simulink model "delay_plant_2015B"  (R2015b)
settings: Solver=VariableStepAuto  StartTime=0.0  StopTime=sim_run  FixedStep=0.0001  RelTol=1e-3
undefined symbols (not defined in the file): DiscIntNeverNeededParam, Standard_Devices, start_packet_test, UDP_Protocol, zh_step
libraries: sldrtlib x2, simulink x1, dspnetwork x1
settings Model: Creator=Anony  LastModifiedBy=Anony

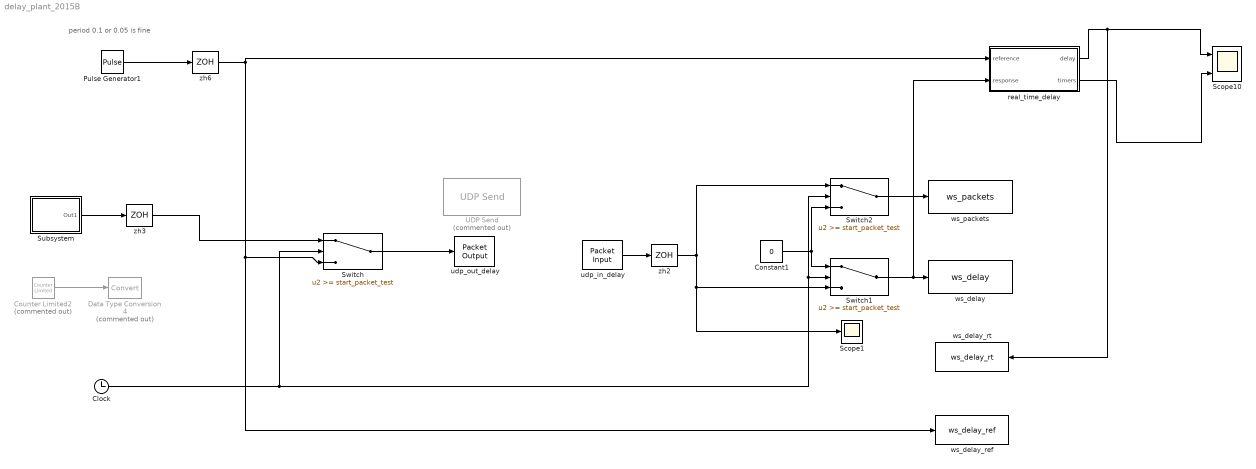
== system delay_plant_2015B ==
  note: period 0.1 or 0.05 is fine
  Clock : Clock
  Constant1 : Constant  Value=0
  Counter Limited2 : simulink/Sources/Counter Limited  Commented=on  uplimit=9999  tsamp=0.001
  Data Type Conversion4 : DataTypeConversion  Commented=on
  Pulse Generator1 : DiscretePulseGenerator  PulseType=Time based  Period=0.5  PulseWidth=0.000001
  Scope1 : Scope
  Scope10 : Scope  NumInputPorts=2
  Subsystem : Subsystem
  Switch : Switch  Threshold=start_packet_test
  Switch1 : Switch  Threshold=start_packet_test
  Switch2 : Switch  Threshold=start_packet_test
  UDP Send : dspnetwork/UDP Send  Commented=on  remoteURL='127.0.0.1'  remotePort=25000  localURL='0.0.0.0'  localPortSource=Automatically determine  localPort=-1  sampletime=-1  separateLengthPort=0
  real_time_delay : Subsystem
  udp_in_delay : sldrtlib/Packet Input  SampleTime=0.0001  MaxMissedTicks=inf  ShowMissedTicks=off  YieldWhenWaiting=off  DrvName=Standard_Devices/UDP_Protocol  DrvAddress=27000  DrvOptions=[2468394752 27000]  PacketSize=8  DataTypes='double'  ShowReady=off  ShowError=off  PacketID=1  ByteOrder=1  ShowTimestamp=off
      settings: AttributesFormatString=Standard Devices\nUDP Protocol [6982h]
  udp_out_delay : sldrtlib/Packet Output  SampleTime=0.001  MaxMissedTicks=inf  ShowMissedTicks=off  YieldWhenWaiting=off  DrvName=Standard_Devices/UDP_Protocol  DrvAddress=28000  DrvOptions=[2468394752 28000]  PacketSize=8  DataTypes='double'  ShowReady=off  ShowError=off  PacketID=1  ByteOrder=1  InitialValue=[]  FinalValue=[]
      settings: AttributesFormatString=Standard Devices\nUDP Protocol [6D6Ah]
  ws_delay : ToWorkspace  VariableName=ws_delay  SaveFormat=Timeseries  SampleTime=zh_step
  ws_delay_ref : ToWorkspace  VariableName=ws_delay_ref  SaveFormat=Timeseries  SampleTime=zh_step
  ws_delay_rt : ToWorkspace  VariableName=ws_delay_rt  SaveFormat=Timeseries  SampleTime=zh_step
  ws_packets : ToWorkspace  VariableName=ws_packets  SaveFormat=Timeseries  SampleTime=zh_step
  zh2 : ZeroOrderHold  SampleTime=zh_step
  zh3 : ZeroOrderHold  SampleTime=0.001
  zh6 : ZeroOrderHold  SampleTime=zh_step
  wires:
  udp_in_delay/1 -> zh2/1
  zh6/1 -> Switch/3, ws_delay_ref/1, real_time_delay/1(reference)
  zh2/1 -> Switch2/1, Scope1/1, Switch1/3
  real_time_delay/1(delay) -> ws_delay_rt/1, Scope10/1
  real_time_delay/2(timers) -> Scope10/2
  Pulse Generator1/1 -> zh6/1
  Subsystem/1(Out1) -> zh3/1
  zh3/1 -> Switch/1
  Switch/1 -> udp_out_delay/1
  Clock/1 -> Switch2/2, Switch1/2, Switch/2
  Counter Limited2/1 -> Data Type Conversion4/1
  Switch1/1 -> real_time_delay/2(response), ws_delay/1
  Constant1/1 -> Switch2/3, Switch1/1
  Switch2/1 -> ws_packets/1

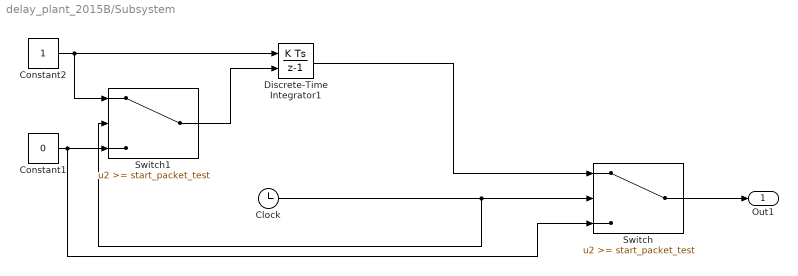
== system delay_plant_2015B/Subsystem ==
  Clock : Clock
  Constant1 : Constant  Value=0
  Constant2 : Constant
  Discrete-Time Integrator1 : DiscreteIntegrator  gainval=1000  ExternalReset=rising  InitialConditionSetting=State (most efficient)  SampleTime=0.001  ICPrevOutput=DiscIntNeverNeededParam  ICPrevScaledInput=DiscIntNeverNeededParam
  Switch : Switch  Threshold=start_packet_test
  Switch1 : Switch  Threshold=start_packet_test
  Out1 : Outport
  wires:
  Discrete-Time Integrator1/1 -> Switch/1
  Constant2/1 -> Discrete-Time Integrator1/1, Switch1/1
  Constant1/1 -> Switch/3, Switch1/3
  Switch/1 -> Out1/1
  Clock/1 -> Switch1/2, Switch/2
  Switch1/1 -> Discrete-Time Integrator1/2

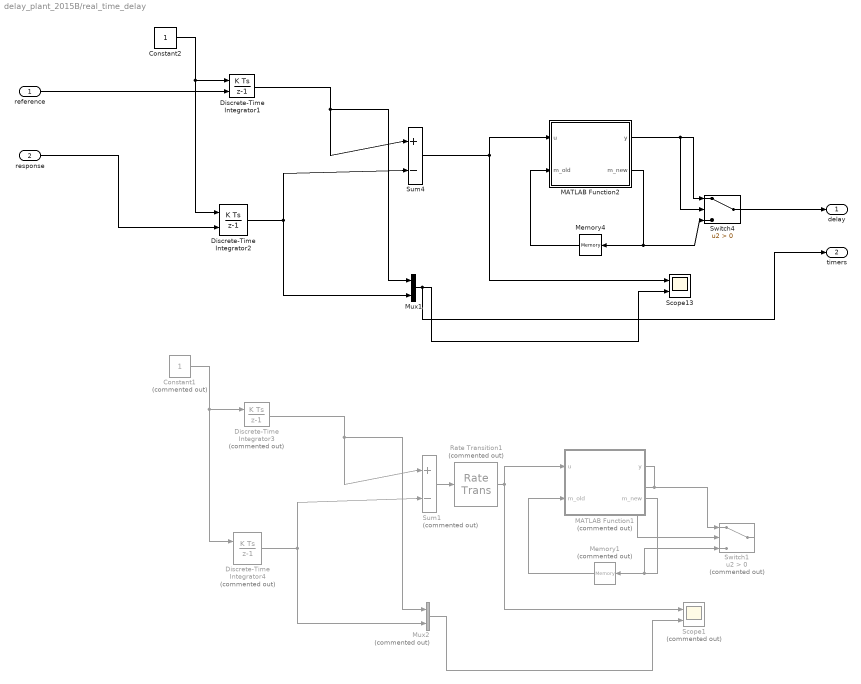
== system delay_plant_2015B/real_time_delay ==
  reference : Inport
  response : Inport  Port=2
  Constant1 : Constant  Commented=on
  Constant2 : Constant
  Discrete-Time Integrator1 : DiscreteIntegrator  ExternalReset=rising  InitialConditionSetting=State (most efficient)  SampleTime=0.001  ICPrevOutput=DiscIntNeverNeededParam  ICPrevScaledInput=DiscIntNeverNeededParam
  Discrete-Time Integrator2 : DiscreteIntegrator  ExternalReset=rising  InitialConditionSetting=State (most efficient)  SampleTime=0.001  ICPrevOutput=DiscIntNeverNeededParam  ICPrevScaledInput=DiscIntNeverNeededParam
  Discrete-Time Integrator3 : DiscreteIntegrator  Commented=on  ExternalReset=rising  InitialConditionSetting=State (most efficient)  SampleTime=0.001  ICPrevOutput=DiscIntNeverNeededParam  ICPrevScaledInput=DiscIntNeverNeededParam
  Discrete-Time Integrator4 : DiscreteIntegrator  Commented=on  ExternalReset=rising  InitialConditionSetting=State (most efficient)  SampleTime=0.001  ICPrevOutput=DiscIntNeverNeededParam  ICPrevScaledInput=DiscIntNeverNeededParam
  MATLAB Function1 : MATLAB Function  Commented=on  TreatAsAtomicUnit=on
  MATLAB Function2 : MATLAB Function  TreatAsAtomicUnit=on
  Memory1 : Memory  Commented=on
  Memory4 : Memory
  Mux1 : Mux  Inputs=2
  Mux2 : Mux  Commented=on  Inputs=2
  Rate Transition1 : RateTransition  Commented=on  OutPortSampleTimeOpt=Inherit
  Scope1 : Scope  Commented=on  NumInputPorts=2
  Scope13 : Scope  NumInputPorts=2
  Sum1 : Sum  Commented=on  Inputs=|+-
  Sum4 : Sum  Inputs=|+-
  Switch1 : Switch  Commented=on  Criteria=u2 > Threshold
  Switch4 : Switch  Criteria=u2 > Threshold
  delay : Outport
  timers : Outport  Port=2
  wires:
  Discrete-Time Integrator1/1 -> Mux1/1, Sum4/1
  reference/1 -> Discrete-Time Integrator1/2
  Constant2/1 -> Discrete-Time Integrator2/1, Discrete-Time Integrator1/1
  response/1 -> Discrete-Time Integrator2/2
  Switch4/1 -> delay/1
  MATLAB Function2/2(m_new) -> Memory4/1, Switch4/3
  Memory4/1 -> MATLAB Function2/2(m_old)
  Discrete-Time Integrator2/1 -> Mux1/2, Sum4/2
  Mux1/1 -> timers/1, Scope13/2
  MATLAB Function2/1(y) -> Switch4/2, Switch4/1
  Sum4/1 -> Scope13/1, MATLAB Function2/1(u)
  Discrete-Time Integrator3/1 -> Sum1/1, Mux2/1
  Constant1/1 -> Discrete-Time Integrator3/1, Discrete-Time Integrator4/1
  MATLAB Function1/2(m_new) -> Switch1/3, Memory1/1
  Sum1/1 -> Rate Transition1/1
  Memory1/1 -> MATLAB Function1/2(m_old)
  Discrete-Time Integrator4/1 -> Sum1/2, Mux2/2
  Mux2/1 -> Scope1/2
  MATLAB Function1/1(y) -> Switch1/1, Switch1/2
  Rate Transition1/1 -> MATLAB Function1/1(u), Scope1/1

== matlab function delay_plant_2015B/real_time_delay/MATLAB Function1 ==
  data: u input; y output; m_new output; m_old input
function [y,m_new] = fcn(u,m_old)
%#codegen
if(u>0)
    y = u;
    m_new = u;
else
    y =0;
    m_new = m_old;
end

== matlab function delay_plant_2015B/real_time_delay/MATLAB Function2 ==
  data: u input; y output; m_new output; m_old input
function [y,m_new] = fcn(u,m_old)
%#codegen
if(u>0)
    y = u;
    m_new = u;
else
    y =0;
    m_new = m_old;
end
